simulink model "PrintingPID"  (R2020b)
settings: Solver=ode45  StartTime=0.0  StopTime=2.5  RelTol=1e-3
undefined symbols (not defined in the file or in its folder): daq, drv, est_par, gbox, io, mech, mld, mot, pid, rads2rpm, rpm2degs, sens
libraries: simulink x2
settings Model: Creator=Utente  LastModifiedBy=Utente
settings SolverCC: ZeroCrossAlgorithm=Adaptive
settings DataIOCC: ReturnWorkspaceOutputs=off
settings DebuggingCC: IgnoredZcDiagnostic=none

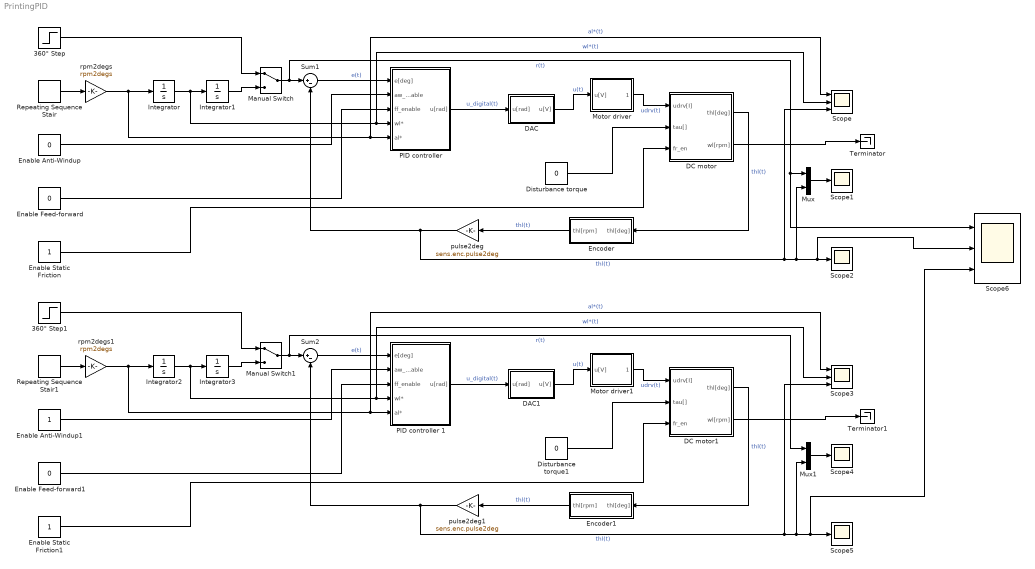
== system PrintingPID ==
  360° Step : Step  Time=0  After=360  SampleTime=0
  360° Step1 : Step  Time=0  After=360  SampleTime=0
  DAC : Subsystem
  DAC1 : Subsystem
  DC motor : Subsystem
  DC motor1 : Subsystem
  Disturbance torque : Constant  Value=0
  Disturbance torque1 : Constant  Value=0
  Enable Anti-Windup : Constant  Value=0
  Enable Anti-Windup1 : Constant
  Enable Feed-forward : Constant  Value=0
  Enable Feed-forward1 : Constant  Value=0
  Enable Static Friction : Constant
  Enable Static Friction1 : Constant
  Encoder : Subsystem
  Encoder1 : Subsystem
  Integrator{,1..3} (4 alike) : Integrator
  Manual Switch : ManualSwitch
  Manual Switch1 : ManualSwitch
  Motor driver : Subsystem
  Motor driver1 : Subsystem
  Mux : Mux  Inputs=2
  Mux1 : Mux  Inputs=2
  "PID controller " : Subsystem
  PID controller 1 : Subsystem
  Repeating Sequence Stair : simulink/Sources/Repeating Sequence Stair  OutValues=[900 0 -900 -900 0 900].'  tsamp=0.5  OutMin=[]  OutMax=[]  OutDataTypeStr=double  OutputDataTypeScalingMode=double  OutDataType=fixdt(0,8)  ConRadixGroup=Best Precision: Vector-wise  OutScaling=2^-12
  Repeating Sequence Stair1 : simulink/Sources/Repeating Sequence Stair  OutValues=[900 0 -900 -900 0 900].'  tsamp=0.5  OutMin=[]  OutMax=[]  OutDataTypeStr=double  OutputDataTypeScalingMode=double  OutDataType=fixdt(0,8)  ConRadixGroup=Best Precision: Vector-wise  OutScaling=2^-12
  Scope : Scope  NumInputPorts=3
  Scope{1..2,4..5} (4 alike) : Scope
  Scope3 : Scope  NumInputPorts=3
  Scope6 : Scope  NumInputPorts=3
  Sum1 : Sum  Inputs=|+-
  Sum2 : Sum  Inputs=|+-
  Terminator : Terminator
  Terminator1 : Terminator
  pulse2deg : Gain  Gain=sens.enc.pulse2deg
  pulse2deg1 : Gain  Gain=sens.enc.pulse2deg
  rpm2degs : Gain  Gain=rpm2degs
  rpm2degs1 : Gain  Gain=rpm2degs
  wires:
  Motor driver/1(udrv[I]) -> DC motor/1(udrv[I])  "udrv(t)"
  DAC/1(u[V]) -> Motor driver/1(u[V])  "u(t)"
  Encoder/1(thl[rpm]) -> pulse2deg/1  "thl(t)"
  pulse2deg/1 -> Scope/3, Mux/2, Scope6/2, Scope2/1, Sum1/2  "thl(t)"
  Sum1/1 -> "PID controller "/1(e[deg])  "e(t)"
  "PID controller "/1(u[rad]) -> DAC/1(u[rad])  "u_digital(t)"
  DC motor/1(thl[deg]) -> Encoder/1(thl[deg])  "thl(t)"
  360° Step/1 -> Manual Switch/1
  Disturbance torque/1 -> DC motor/2(tau[])
  Enable Anti-Windup/1 -> "PID controller "/2(aw_enable)
  Manual Switch/1 -> Scope6/1, Mux/1, Sum1/1  "r(t)"
  Enable Feed-forward/1 -> "PID controller "/3(ff_enable)
  Repeating Sequence Stair/1 -> rpm2degs/1
  rpm2degs/1 -> Scope/1, "PID controller "/5(al*), Integrator/1  "al*(t)"
  Integrator1/1 -> Manual Switch/2
  Integrator/1 -> Scope/2, "PID controller "/4(wl*), Integrator1/1  "wl*(t)"
  Mux/1 -> Scope1/1
  DC motor/2(wl[rpm]) -> Terminator/1
  Enable Static Friction/1 -> DC motor/3(fr_en)
  Motor driver1/1(udrv[I]) -> DC motor1/1(udrv[I])  "udrv(t)"
  360° Step1/1 -> Manual Switch1/1
  rpm2degs1/1 -> Scope3/1, PID controller 1/5(al*), Integrator2/1  "al*(t)"
  DAC1/1(u[V]) -> Motor driver1/1(u[V])  "u(t)"
  Sum2/1 -> PID controller 1/1(e[deg])  "e(t)"
  Mux1/1 -> Scope4/1
  Disturbance torque1/1 -> DC motor1/2(tau[])
  Integrator2/1 -> Scope3/2, PID controller 1/4(wl*), Integrator3/1  "wl*(t)"
  Integrator3/1 -> Manual Switch1/2
  Repeating Sequence Stair1/1 -> rpm2degs1/1
  Enable Static Friction1/1 -> DC motor1/3(fr_en)
  PID controller 1/1(u[rad]) -> DAC1/1(u[rad])  "u_digital(t)"
  Enable Anti-Windup1/1 -> PID controller 1/2(aw_enable)
  DC motor1/2(wl[rpm]) -> Terminator1/1
  Manual Switch1/1 -> Mux1/1, Sum2/1  "r(t)"
  Enable Feed-forward1/1 -> PID controller 1/3(ff_enable)
  DC motor1/1(thl[deg]) -> Encoder1/1(thl[deg])  "thl(t)"
  pulse2deg1/1 -> Scope3/3, Mux1/2, Scope6/3, Scope5/1, Sum2/2  "thl(t)"
  Encoder1/1(thl[rpm]) -> pulse2deg1/1  "thl(t)"

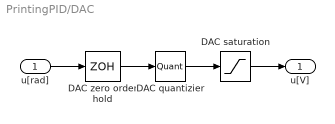
== system PrintingPID/DAC ==
  u[rad] : Inport
  DAC quantizier : Quantizer  QuantizationInterval=daq.dac.q
  DAC saturation : Saturate  UpperLimit=daq.dac.vdd  LowerLimit=daq.dac.vss
  DAC zero order hold : ZeroOrderHold  SampleTime=daq.dac.T_s
  u[V] : Outport
  wires:
  DAC quantizier/1 -> DAC saturation/1
  DAC zero order hold/1 -> DAC quantizier/1
  DAC saturation/1 -> u[V]/1
  u[rad]/1 -> DAC zero order hold/1

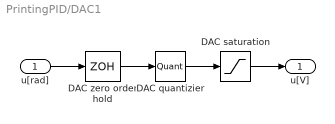
== system PrintingPID/DAC1 ==
  u[rad] : Inport
  DAC quantizier : Quantizer  QuantizationInterval=daq.dac.q
  DAC saturation : Saturate  UpperLimit=daq.dac.vdd  LowerLimit=daq.dac.vss
  DAC zero order hold : ZeroOrderHold  SampleTime=daq.dac.T_s
  u[V] : Outport
  wires:
  DAC quantizier/1 -> DAC saturation/1
  DAC zero order hold/1 -> DAC quantizier/1
  DAC saturation/1 -> u[V]/1
  u[rad]/1 -> DAC zero order hold/1

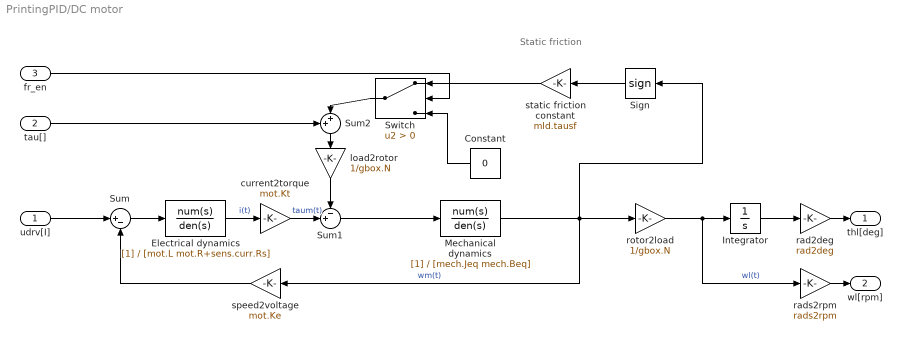
== system PrintingPID/DC motor ==
  note: Static friction
  udrv[I] : Inport  Unit=V
  tau[] : Inport  Port=2  Unit=V
  fr_en : Inport  Port=3  Unit=V
  Constant : Constant  Value=0
  Electrical dynamics : TransferFcn  Denominator=[mot.L mot.R+sens.curr.Rs]
  Integrator : Integrator
  Mechanical dynamics : TransferFcn  Denominator=[mech.Jeq mech.Beq]
  Sign : Signum  ZeroCross=off
  Sum : Sum  Inputs=|+-
  Sum1 : Sum  Inputs=-+|
  Sum2 : Sum  Inputs=++|
  Switch : Switch  Criteria=u2 > Threshold
  current2torque : Gain  Gain=mot.Kt
  load2rotor : Gain  Gain=1/gbox.N
  rad2deg : Gain  Gain=rad2deg
  rads2rpm : Gain  Gain=rads2rpm
  rotor2load : Gain  Gain=1/gbox.N
  speed2voltage : Gain  Gain=mot.Ke
  static friction constant : Gain  Gain=mld.tausf
  thl[deg] : Outport  Unit=deg
  wl[rpm] : Outport  Port=2  Unit=rpm
  wires:
  load2rotor/1 -> Sum1/1
  Mechanical dynamics/1 -> Sign/1, rotor2load/1, speed2voltage/1  "wm(t)"
  Sign/1 -> static friction constant/1
  current2torque/1 -> Sum1/2  "taum(t)"
  Sum1/1 -> Mechanical dynamics/1
  speed2voltage/1 -> Sum/2
  rotor2load/1 -> rads2rpm/1, Integrator/1  "wl(t)"
  Electrical dynamics/1 -> current2torque/1  "i(t)"
  Integrator/1 -> rad2deg/1
  Sum/1 -> Electrical dynamics/1
  rads2rpm/1 -> wl[rpm]/1
  rad2deg/1 -> thl[deg]/1
  udrv[I]/1 -> Sum/1
  Sum2/1 -> load2rotor/1
  tau[]/1 -> Sum2/1
  static friction constant/1 -> Switch/1
  Switch/1 -> Sum2/2
  Constant/1 -> Switch/3
  fr_en/1 -> Switch/2

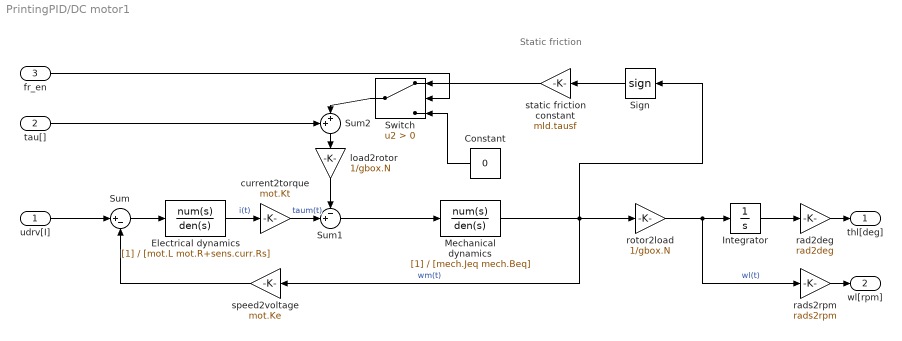
== system PrintingPID/DC motor1 ==
  note: Static friction
  udrv[I] : Inport  Unit=V
  tau[] : Inport  Port=2  Unit=V
  fr_en : Inport  Port=3  Unit=V
  Constant : Constant  Value=0
  Electrical dynamics : TransferFcn  Denominator=[mot.L mot.R+sens.curr.Rs]
  Integrator : Integrator
  Mechanical dynamics : TransferFcn  Denominator=[mech.Jeq mech.Beq]
  Sign : Signum  ZeroCross=off
  Sum : Sum  Inputs=|+-
  Sum1 : Sum  Inputs=-+|
  Sum2 : Sum  Inputs=++|
  Switch : Switch  Criteria=u2 > Threshold
  current2torque : Gain  Gain=mot.Kt
  load2rotor : Gain  Gain=1/gbox.N
  rad2deg : Gain  Gain=rad2deg
  rads2rpm : Gain  Gain=rads2rpm
  rotor2load : Gain  Gain=1/gbox.N
  speed2voltage : Gain  Gain=mot.Ke
  static friction constant : Gain  Gain=mld.tausf
  thl[deg] : Outport  Unit=deg
  wl[rpm] : Outport  Port=2  Unit=rpm
  wires:
  load2rotor/1 -> Sum1/1
  Mechanical dynamics/1 -> Sign/1, rotor2load/1, speed2voltage/1  "wm(t)"
  Sign/1 -> static friction constant/1
  current2torque/1 -> Sum1/2  "taum(t)"
  Sum1/1 -> Mechanical dynamics/1
  speed2voltage/1 -> Sum/2
  rotor2load/1 -> rads2rpm/1, Integrator/1  "wl(t)"
  Electrical dynamics/1 -> current2torque/1  "i(t)"
  Integrator/1 -> rad2deg/1
  Sum/1 -> Electrical dynamics/1
  rads2rpm/1 -> wl[rpm]/1
  rad2deg/1 -> thl[deg]/1
  udrv[I]/1 -> Sum/1
  Sum2/1 -> load2rotor/1
  tau[]/1 -> Sum2/1
  static friction constant/1 -> Switch/1
  Switch/1 -> Sum2/2
  Constant/1 -> Switch/3
  fr_en/1 -> Switch/2

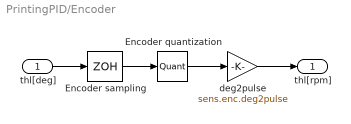
== system PrintingPID/Encoder ==
  thl[deg] : Inport
  Encoder quantization : Quantizer  QuantizationInterval=sens.enc.q
  Encoder sampling : ZeroOrderHold  SampleTime=sens.enc.T_s
  deg2pulse : Gain  Gain=sens.enc.deg2pulse
  thl[rpm] : Outport
  wires:
  Encoder quantization/1 -> deg2pulse/1
  deg2pulse/1 -> thl[rpm]/1
  Encoder sampling/1 -> Encoder quantization/1
  thl[deg]/1 -> Encoder sampling/1

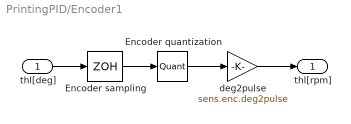
== system PrintingPID/Encoder1 ==
  thl[deg] : Inport
  Encoder quantization : Quantizer  QuantizationInterval=sens.enc.q
  Encoder sampling : ZeroOrderHold  SampleTime=sens.enc.T_s
  deg2pulse : Gain  Gain=sens.enc.deg2pulse
  thl[rpm] : Outport
  wires:
  Encoder quantization/1 -> deg2pulse/1
  deg2pulse/1 -> thl[rpm]/1
  Encoder sampling/1 -> Encoder quantization/1
  thl[deg]/1 -> Encoder sampling/1

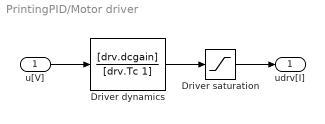
== system PrintingPID/Motor driver ==
  u[V] : Inport
  Driver dynamics : TransferFcn  Numerator=[drv.dcgain]  Denominator=[drv.Tc 1]
  Driver saturation : Saturate  UpperLimit=drv.vp  LowerLimit=drv.vm
  udrv[I] : Outport
  wires:
  Driver saturation/1 -> udrv[I]/1
  Driver dynamics/1 -> Driver saturation/1
  u[V]/1 -> Driver dynamics/1

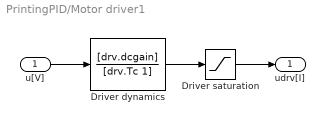
== system PrintingPID/Motor driver1 ==
  u[V] : Inport
  Driver dynamics : TransferFcn  Numerator=[drv.dcgain]  Denominator=[drv.Tc 1]
  Driver saturation : Saturate  UpperLimit=drv.vp  LowerLimit=drv.vm
  udrv[I] : Outport
  wires:
  Driver saturation/1 -> udrv[I]/1
  Driver dynamics/1 -> Driver saturation/1
  u[V]/1 -> Driver dynamics/1

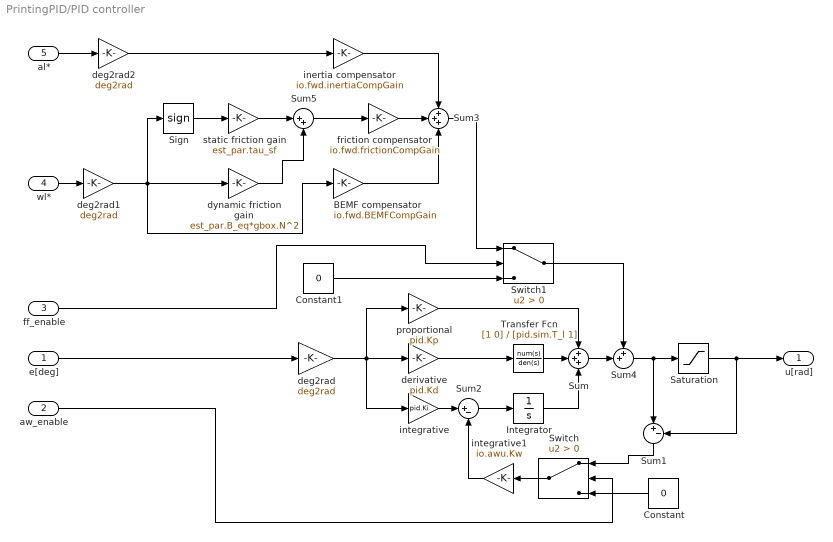
== system PrintingPID/PID controller  ==
  e[deg] : Inport  Unit=deg
  aw_enable : Inport  Port=2  Unit=deg
  ff_enable : Inport  Port=3  Unit=deg
  wl* : Inport  Port=4  Unit=deg
  al* : Inport  Port=5  Unit=deg
  BEMF compensator : Gain  Gain=io.fwd.BEMFCompGain
  Constant : Constant  Value=0
  Constant1 : Constant  Value=0
  Integrator : Integrator
  Saturation : Saturate  UpperLimit=daq.dac.vdd  LowerLimit=daq.dac.vss
  Sign : Signum
  Sum : Sum  Inputs=+++
  Sum1 : Sum  Inputs=|+-
  Sum2 : Sum  Inputs=|+-
  Sum3 : Sum  Inputs=+++
  Sum4 : Sum  Inputs=++|
  Sum5 : Sum  Inputs=|++
  Switch : Switch  Criteria=u2 > Threshold
  Switch1 : Switch  Criteria=u2 > Threshold
  Transfer Fcn : TransferFcn  Numerator=[1 0]  Denominator=[pid.sim.T_l 1]
  deg2rad : Gain  Gain=deg2rad
  deg2rad1 : Gain  Gain=deg2rad
  deg2rad2 : Gain  Gain=deg2rad
  derivative : Gain  Gain=pid.Kd
  dynamic friction gain : Gain  Gain=est_par.B_eq*gbox.N^2
  friction compensator : Gain  Gain=io.fwd.frictionCompGain
  inertia compensator : Gain  Gain=io.fwd.inertiaCompGain
  integrative : Gain  Gain=pid.Ki
  integrative1 : Gain  Gain=io.awu.Kw
  proportional : Gain  Gain=pid.Kp
  static friction gain : Gain  Gain=est_par.tau_sf
  u[rad] : Outport
  wires:
  deg2rad/1 -> integrative/1, derivative/1, proportional/1
  proportional/1 -> Sum/1
  Saturation/1 -> Sum1/2, u[rad]/1
  integrative/1 -> Sum2/1
  Sum2/1 -> Integrator/1
  integrative1/1 -> Sum2/2
  Integrator/1 -> Sum/3
  Transfer Fcn/1 -> Sum/2
  derivative/1 -> Transfer Fcn/1
  aw_enable/1 -> Switch/2
  Constant/1 -> Switch/3
  Switch/1 -> integrative1/1
  Sum1/1 -> Switch/1
  ff_enable/1 -> Switch1/2
  Constant1/1 -> Switch1/3
  friction compensator/1 -> Sum3/2
  inertia compensator/1 -> Sum3/1
  BEMF compensator/1 -> Sum3/3
  Sum4/1 -> Saturation/1, Sum1/1
  Sign/1 -> static friction gain/1
  static friction gain/1 -> Sum5/1
  dynamic friction gain/1 -> Sum5/2
  Sum5/1 -> friction compensator/1
  al*/1 -> deg2rad2/1
  wl*/1 -> deg2rad1/1
  Sum3/1 -> Switch1/1
  Sum/1 -> Sum4/2
  Switch1/1 -> Sum4/1
  deg2rad1/1 -> BEMF compensator/1, Sign/1, dynamic friction gain/1
  deg2rad2/1 -> inertia compensator/1
  e[deg]/1 -> deg2rad/1

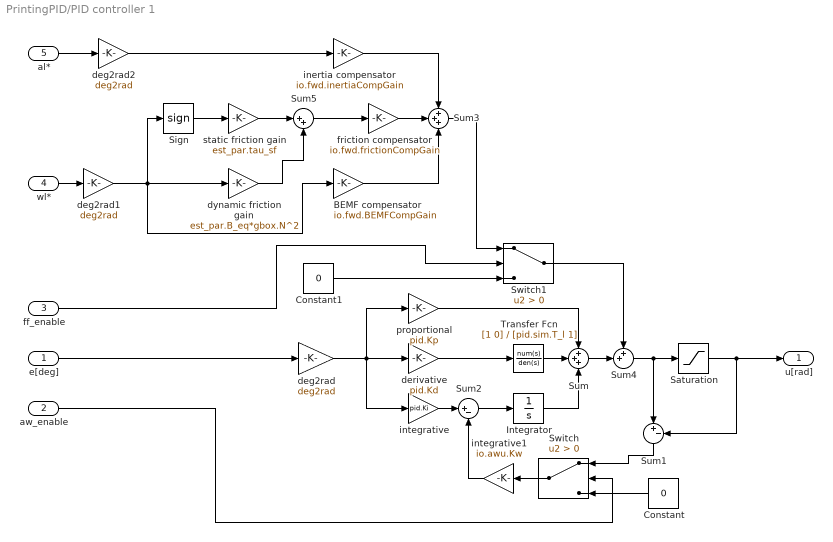
== system PrintingPID/PID controller 1 ==
  e[deg] : Inport  Unit=deg
  aw_enable : Inport  Port=2  Unit=deg
  ff_enable : Inport  Port=3  Unit=deg
  wl* : Inport  Port=4  Unit=deg
  al* : Inport  Port=5  Unit=deg
  BEMF compensator : Gain  Gain=io.fwd.BEMFCompGain
  Constant : Constant  Value=0
  Constant1 : Constant  Value=0
  Integrator : Integrator
  Saturation : Saturate  UpperLimit=daq.dac.vdd  LowerLimit=daq.dac.vss
  Sign : Signum
  Sum : Sum  Inputs=+++
  Sum1 : Sum  Inputs=|+-
  Sum2 : Sum  Inputs=|+-
  Sum3 : Sum  Inputs=+++
  Sum4 : Sum  Inputs=++|
  Sum5 : Sum  Inputs=|++
  Switch : Switch  Criteria=u2 > Threshold
  Switch1 : Switch  Criteria=u2 > Threshold
  Transfer Fcn : TransferFcn  Numerator=[1 0]  Denominator=[pid.sim.T_l 1]
  deg2rad : Gain  Gain=deg2rad
  deg2rad1 : Gain  Gain=deg2rad
  deg2rad2 : Gain  Gain=deg2rad
  derivative : Gain  Gain=pid.Kd
  dynamic friction gain : Gain  Gain=est_par.B_eq*gbox.N^2
  friction compensator : Gain  Gain=io.fwd.frictionCompGain
  inertia compensator : Gain  Gain=io.fwd.inertiaCompGain
  integrative : Gain  Gain=pid.Ki
  integrative1 : Gain  Gain=io.awu.Kw
  proportional : Gain  Gain=pid.Kp
  static friction gain : Gain  Gain=est_par.tau_sf
  u[rad] : Outport
  wires:
  deg2rad/1 -> integrative/1, derivative/1, proportional/1
  proportional/1 -> Sum/1
  Saturation/1 -> Sum1/2, u[rad]/1
  integrative/1 -> Sum2/1
  Sum2/1 -> Integrator/1
  integrative1/1 -> Sum2/2
  Integrator/1 -> Sum/3
  Transfer Fcn/1 -> Sum/2
  derivative/1 -> Transfer Fcn/1
  aw_enable/1 -> Switch/2
  Constant/1 -> Switch/3
  Switch/1 -> integrative1/1
  Sum1/1 -> Switch/1
  ff_enable/1 -> Switch1/2
  Constant1/1 -> Switch1/3
  friction compensator/1 -> Sum3/2
  inertia compensator/1 -> Sum3/1
  BEMF compensator/1 -> Sum3/3
  Sum4/1 -> Saturation/1, Sum1/1
  Sign/1 -> static friction gain/1
  static friction gain/1 -> Sum5/1
  dynamic friction gain/1 -> Sum5/2
  Sum5/1 -> friction compensator/1
  al*/1 -> deg2rad2/1
  wl*/1 -> deg2rad1/1
  Sum3/1 -> Switch1/1
  Sum/1 -> Sum4/2
  Switch1/1 -> Sum4/1
  deg2rad1/1 -> BEMF compensator/1, Sign/1, dynamic friction gain/1
  deg2rad2/1 -> inertia compensator/1
  e[deg]/1 -> deg2rad/1
